simulink model "boostsim"  (R2020a)
settings: Solver=FixedStepAuto  StartTime=0.0  StopTime=0.4  FixedStep=1e-5  RelTol=1e-3
undefined symbols (not defined in the file or in its folder): G
libraries: cstblocks x8
settings Model: Creator=Laza  LastModifiedBy=Laza

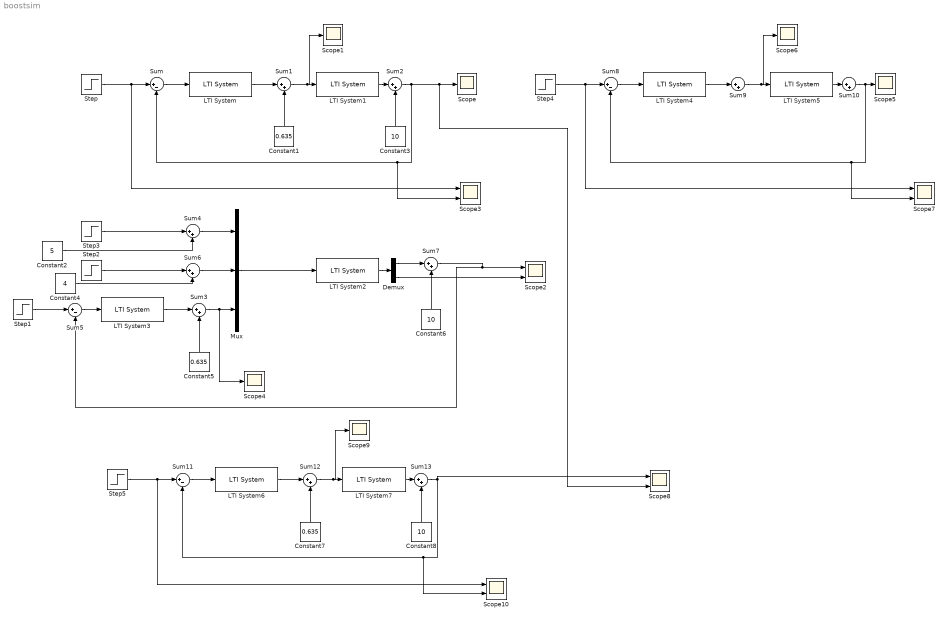
== system boostsim ==
  Constant1 : Constant  Value=0.635
  Constant2 : Constant  Value=5
  Constant3 : Constant  Value=10
  Constant4 : Constant  Value=4
  Constant5 : Constant  Value=0.635
  Constant6 : Constant  Value=10
  Constant7 : Constant  Value=0.635
  Constant8 : Constant  Value=10
  Demux : Demux  Outputs=2
  LTI System : cstblocks/LTI System  sys=K  IC=[]
  LTI System1 : cstblocks/LTI System  sys=G(3)  IC=[]
  LTI System2 : cstblocks/LTI System  sys=Hs  IC=[]
  LTI System3 : cstblocks/LTI System  sys=K  IC=[]
  LTI System4 : cstblocks/LTI System  sys=K  IC=[]
  LTI System5 : cstblocks/LTI System  sys=G(3)  IC=[]
  LTI System6 : cstblocks/LTI System  sys=Gcomp  IC=[]
  LTI System7 : cstblocks/LTI System  sys=G(3)  IC=[]
  Mux : Mux  Inputs=3
  Scope{,1,4..6,9} (6 alike) : Scope
  Scope{2..3,7..8,10} (5 alike) : Scope  NumInputPorts=2
  Step{,1,4..5} (4 alike) : Step  Time=0.1  Before=10  After=12  SampleTime=0
  Step2 : Step  Time=0.2  After=-1  SampleTime=0
  Step3 : Step  Time=0.3  SampleTime=0
  Sum{,5,8,11} (4 alike) : Sum  Inputs=|+-
  Sum{1..4,6..7,9..10,12..13} (10 alike) : Sum  Inputs=|++
  wires:
  Sum/1 -> LTI System/1
  Step/1 -> Scope3/1, Sum/1
  Constant1/1 -> Sum1/2
  LTI System1/1 -> Sum2/1
  Sum1/1 -> Scope1/1, LTI System1/1
  LTI System/1 -> Sum1/1
  Constant3/1 -> Sum2/2
  Sum2/1 -> Scope8/2, Scope/1, Scope3/2, Sum/2
  LTI System2/1 -> Demux/1
  Mux/1 -> LTI System2/1
  Constant5/1 -> Sum3/2
  Sum3/1 -> Scope4/1, Mux/3
  Sum5/1 -> LTI System3/1
  Step1/1 -> Sum5/1
  Constant4/1 -> Sum6/2
  Sum6/1 -> Mux/2
  Demux/2 -> Scope2/2
  LTI System3/1 -> Sum3/1
  Step2/1 -> Sum6/1
  Constant2/1 -> Sum4/2
  Sum4/1 -> Mux/1
  Step3/1 -> Sum4/1
  Constant6/1 -> Sum7/2
  Demux/1 -> Sum7/1
  Sum7/1 -> Sum5/2, Scope2/1
  Sum10/1 -> Sum8/2, Scope7/2, Scope5/1
  LTI System4/1 -> Sum9/1
  Sum9/1 -> LTI System5/1, Scope6/1
  LTI System5/1 -> Sum10/1
  Step4/1 -> Sum8/1, Scope7/1
  Sum8/1 -> LTI System4/1
  Sum13/1 -> Sum11/2, Scope10/2, Scope8/1
  Constant8/1 -> Sum13/2
  LTI System6/1 -> Sum12/1
  Sum12/1 -> LTI System7/1, Scope9/1
  LTI System7/1 -> Sum13/1
  Constant7/1 -> Sum12/2
  Step5/1 -> Sum11/1, Scope10/1
  Sum11/1 -> LTI System6/1
